simulink model "Week2_Problem1"  (R2020a)
settings: Solver=VariableStepAuto  StartTime=0.0  StopTime=10.0  RelTol=1e-3
settings Model: Creator=tnradm  LastModifiedBy=tnradm

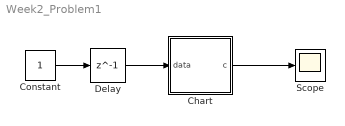
== system Week2_Problem1 ==
  Chart : Stateflow chart  TreatAsAtomicUnit=on
  Constant : Constant
  Delay : Delay  DelayLength=1
  Scope : Scope
  wires:
  Constant/1 -> Delay/1
  Delay/1 -> Chart/1(data)
  Chart/1(c) -> Scope/1

== stateflow chart Week2_Problem1/Chart ==
  state reset
    entry:c=0;
  state counter
    entry:
  state incremend
    entry:c=c+1;
  (default) -> counter : {c=data}
  reset -> counter
  incremend -> reset [order 2] : [c>=5]
  counter -> incremend : [c<5]
  incremend -> counter [order 1] : [c<5]
  data: data input; c output
